simulink model "pipeline"  (Simulink 10.0)
settings: Solver=VariableStepAuto  StartTime=0.0  StopTime=10000*(1/2e7)  FixedStep=1e-9  RelTol=1e-3
values from neighbouring files (symbols this model uses):
  fsig = 13e6    (= 13000000)    [Pipeline_m.m]
  Ts = ts    (= 1e-08)    [Pipeline_m.m]
  vin_amp = vref*10^(-Vsig_dB/20)    (= 1.8)    [Pipeline_m.m]
settings Model: Creator=user  LastModifiedBy=benve
settings DataIOCC: SaveFormat=Dataset  ReturnWorkspaceOutputs=on
settings OptimizationCC: LifeSpan=auto
settings DebuggingCC: UnderspecifiedInitializationDetection=Simplified  MergeDetectMultiDrivingBlocksExec=error  SFUnexpectedBacktrackingDiag=error  SFNoUnconditionalDefaultTransitionDiag=error  SFExecutionAtInitializationDiag=warning  ArithmeticOperatorsInVariantConditions=error
settings HardwareCC: ProdBitPerPointer=64  ProdBitPerSizeT=64  ProdBitPerPtrDiffT=64  ProdLargestAtomicFloat=Float  ProdIntDivRoundTo=Zero  ProdEndianess=LittleEndian  ProdWordSize=64  ProdHWDeviceType=Intel->x86-64 (Windows64)
settings ModelReferenceCC: PropagateSignalLabelsOutOfModel=on
settings SFSimCC: SimUseLocalCustomCode=on
settings RTWCC: RTWUseLocalCustomCode=on
settings CodeAppCC: StateflowObjectComments=off
settings GRTTargetCC: TargetLangStandard=C99 (ISO)  CombineOutputUpdateFcns=on  GRTInterface=off
settings ConfigComp: CovMetricSettings=dwe  CovHtmlReporting=off  CovSaveCumulativeToWorkspaceVar=off  CovSaveSingleToWorkspaceVar=off

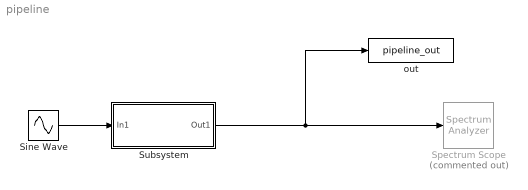
== system pipeline ==
  Sine Wave : Sin  Amplitude=vin_amp  Frequency=2*pi*fsig  SampleTime=Ts  VectorParams1D=off
  Spectrum Scope : SpectrumAnalyzer  Commented=on
  Subsystem : Subsystem  mask{Ts=Ts, vref=1.8}
      mask prompts: Ts "sampling time:"
  out : ToWorkspace  VariableName=pipeline_out  SampleTime=-1
      settings: Save2DSignal=2-D array (concatenate along first dimension)
  wires:
  Sine Wave/1 -> Subsystem/1(In1)
  Subsystem/1(Out1) -> out/1, Spectrum Scope/1

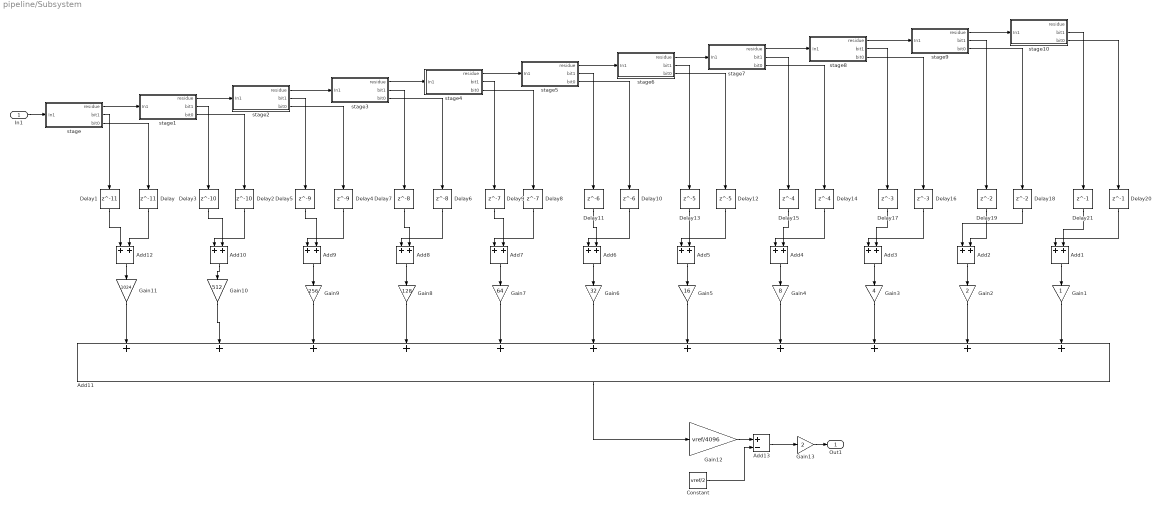
== system pipeline/Subsystem ==
  In1 : Inport
  Add{1..10,12} (11 alike) : Sum
  Add11 : Sum  Inputs=+++++++++++
  Add13 : Sum  Inputs=+-
  Constant : Constant  Value=vref/2
  Delay : Delay  DelayLength=11  SampleTime=Ts
  Delay1 : Delay  DelayLength=11  SampleTime=Ts
  Delay10 : Delay  DelayLength=6  SampleTime=Ts
  Delay11 : Delay  DelayLength=6  SampleTime=Ts
  Delay12 : Delay  DelayLength=5  SampleTime=Ts
  Delay13 : Delay  DelayLength=5  SampleTime=Ts
  Delay14 : Delay  DelayLength=4  SampleTime=Ts
  Delay15 : Delay  DelayLength=4  SampleTime=Ts
  Delay16 : Delay  DelayLength=3  SampleTime=Ts
  Delay17 : Delay  DelayLength=3  SampleTime=Ts
  Delay18 : Delay  SampleTime=Ts
  Delay19 : Delay  SampleTime=Ts
  Delay2 : Delay  DelayLength=10  SampleTime=Ts
  Delay20 : Delay  DelayLength=1  SampleTime=Ts
  Delay21 : Delay  DelayLength=1  SampleTime=Ts
  Delay3 : Delay  DelayLength=10  SampleTime=Ts
  Delay4 : Delay  DelayLength=9  SampleTime=Ts
  Delay5 : Delay  DelayLength=9  SampleTime=Ts
  Delay6 : Delay  DelayLength=8  SampleTime=Ts
  Delay7 : Delay  DelayLength=8  SampleTime=Ts
  Delay8 : Delay  DelayLength=7  SampleTime=Ts
  Delay9 : Delay  DelayLength=7  SampleTime=Ts
  Gain1 : Gain
  Gain10 : Gain  Gain=512
  Gain11 : Gain  Gain=1024
  Gain12 : Gain  Gain=vref/4096
  Gain13 : Gain  Gain=2
  Gain2 : Gain  Gain=2
  Gain3 : Gain  Gain=4
  Gain4 : Gain  Gain=8
  Gain5 : Gain  Gain=16
  Gain6 : Gain  Gain=32
  Gain7 : Gain  Gain=64
  Gain8 : Gain  Gain=128
  Gain9 : Gain  Gain=256
  stage : Subsystem
  stage1 : Subsystem
  stage10 : Subsystem
  stage2 : Subsystem
  stage3 : Subsystem
  stage4 : Subsystem
  stage5 : Subsystem
  stage6 : Subsystem
  stage7 : Subsystem
  stage8 : Subsystem
  stage9 : Subsystem
  Out1 : Outport  VectorParamsAs1DForOutWhenUnconnected=off
  wires:
  stage/1(residue) -> stage1/1(In1)
  stage1/1(residue) -> stage2/1(In1)
  In1/1 -> stage/1(In1)
  stage2/1(residue) -> stage3/1(In1)
  stage3/1(residue) -> stage4/1(In1)
  stage6/1(residue) -> stage7/1(In1)
  stage5/1(residue) -> stage6/1(In1)
  stage4/1(residue) -> stage5/1(In1)
  stage9/1(residue) -> stage10/1(In1)
  stage8/1(residue) -> stage9/1(In1)
  stage7/1(residue) -> stage8/1(In1)
  stage/2(bit1) -> Delay1/1
  stage/3(bit0) -> Delay/1
  stage1/3(bit0) -> Delay2/1
  stage1/2(bit1) -> Delay3/1
  stage2/3(bit0) -> Delay4/1
  stage2/2(bit1) -> Delay5/1
  stage3/2(bit1) -> Delay7/1
  stage3/3(bit0) -> Delay6/1
  stage4/3(bit0) -> Delay8/1
  stage4/2(bit1) -> Delay9/1
  stage5/3(bit0) -> Delay10/1
  stage5/2(bit1) -> Delay11/1
  stage6/2(bit1) -> Delay13/1
  stage6/3(bit0) -> Delay12/1
  stage7/3(bit0) -> Delay14/1
  stage7/2(bit1) -> Delay15/1
  stage8/3(bit0) -> Delay16/1
  stage8/2(bit1) -> Delay17/1
  stage9/2(bit1) -> Delay19/1
  stage9/3(bit0) -> Delay18/1
  stage10/2(bit1) -> Delay21/1
  stage10/3(bit0) -> Delay20/1
  Add1/1 -> Gain1/1
  Delay21/1 -> Add1/2
  Add2/1 -> Gain2/1
  Delay19/1 -> Add2/2
  Delay17/1 -> Add3/2
  Add3/1 -> Gain3/1
  Add4/1 -> Gain4/1
  Delay15/1 -> Add4/2
  Add5/1 -> Gain5/1
  Delay13/1 -> Add5/2
  Add6/1 -> Gain6/1
  Delay11/1 -> Add6/2
  Add7/1 -> Gain7/1
  Delay9/1 -> Add7/2
  Add8/1 -> Gain8/1
  Delay7/1 -> Add8/2
  Add9/1 -> Gain9/1
  Delay5/1 -> Add9/2
  Add10/1 -> Gain10/1
  Delay3/1 -> Add10/2
  Gain1/1 -> Add11/11
  Gain2/1 -> Add11/10
  Gain3/1 -> Add11/9
  Gain4/1 -> Add11/8
  Gain5/1 -> Add11/7
  Gain6/1 -> Add11/6
  Gain7/1 -> Add11/5
  Gain8/1 -> Add11/4
  Gain9/1 -> Add11/3
  Gain10/1 -> Add11/2
  Gain11/1 -> Add11/1
  Delay20/1 -> Add1/1
  Delay18/1 -> Add2/1
  Delay16/1 -> Add3/1
  Delay14/1 -> Add4/1
  Delay12/1 -> Add5/1
  Delay10/1 -> Add6/1
  Delay8/1 -> Add7/1
  Delay6/1 -> Add8/1
  Delay4/1 -> Add9/1
  Delay2/1 -> Add10/1
  Delay1/1 -> Add12/1
  Delay/1 -> Add12/2
  Add12/1 -> Gain11/1
  Add11/1 -> Gain12/1
  Gain12/1 -> Add13/1
  Add13/1 -> Gain13/1
  Constant/1 -> Add13/2
  Gain13/1 -> Out1/1

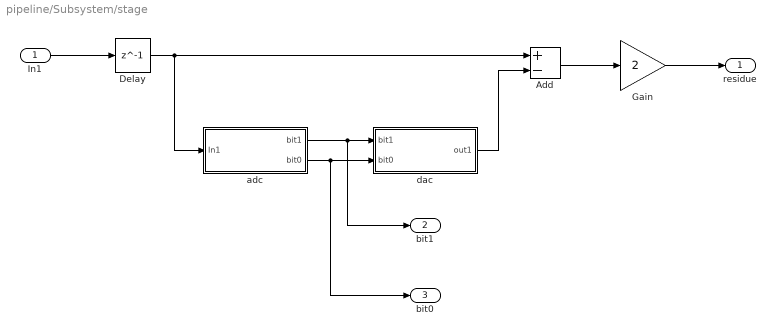
== system pipeline/Subsystem/stage ==
  In1 : Inport
  Add : Sum  Inputs=+-
  Delay : Delay  DelayLength=1  SampleTime=Ts
  Gain : Gain  Gain=2
  adc : Subsystem
  dac : Subsystem
  residue : Outport  VectorParamsAs1DForOutWhenUnconnected=off
  bit1 : Outport  Port=2  VectorParamsAs1DForOutWhenUnconnected=off
  bit0 : Outport  Port=3  VectorParamsAs1DForOutWhenUnconnected=off
  wires:
  adc/1(bit1) -> bit1/1, dac/1(bit1)
  dac/1(out1) -> Add/2
  Delay/1 -> adc/1(In1), Add/1
  Gain/1 -> residue/1
  Add/1 -> Gain/1
  In1/1 -> Delay/1
  adc/2(bit0) -> bit0/1, dac/2(bit0)

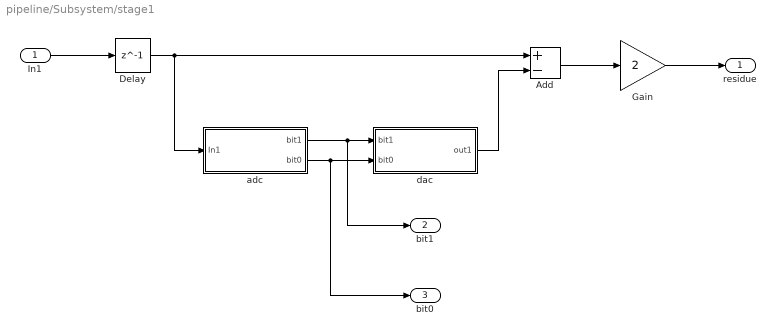
== system pipeline/Subsystem/stage1 ==
  In1 : Inport
  Add : Sum  Inputs=+-
  Delay : Delay  DelayLength=1  SampleTime=Ts
  Gain : Gain  Gain=2
  adc : Subsystem
  dac : Subsystem
  residue : Outport  VectorParamsAs1DForOutWhenUnconnected=off
  bit1 : Outport  Port=2  VectorParamsAs1DForOutWhenUnconnected=off
  bit0 : Outport  Port=3  VectorParamsAs1DForOutWhenUnconnected=off
  wires:
  adc/1(bit1) -> bit1/1, dac/1(bit1)
  dac/1(out1) -> Add/2
  Delay/1 -> adc/1(In1), Add/1
  Gain/1 -> residue/1
  Add/1 -> Gain/1
  In1/1 -> Delay/1
  adc/2(bit0) -> bit0/1, dac/2(bit0)

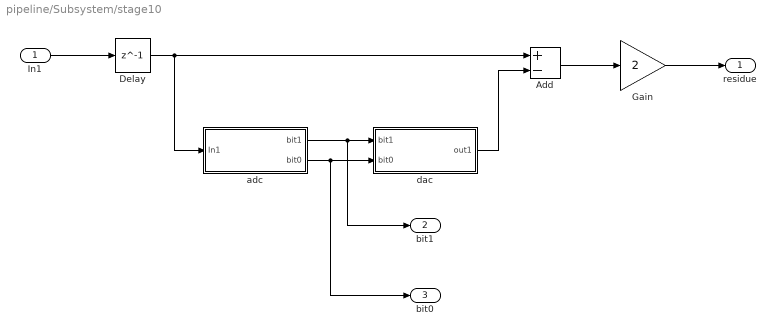
== system pipeline/Subsystem/stage10 ==
  In1 : Inport
  Add : Sum  Inputs=+-
  Delay : Delay  DelayLength=1  SampleTime=Ts
  Gain : Gain  Gain=2
  adc : Subsystem
  dac : Subsystem
  residue : Outport  VectorParamsAs1DForOutWhenUnconnected=off
  bit1 : Outport  Port=2  VectorParamsAs1DForOutWhenUnconnected=off
  bit0 : Outport  Port=3  VectorParamsAs1DForOutWhenUnconnected=off
  wires:
  adc/1(bit1) -> bit1/1, dac/1(bit1)
  dac/1(out1) -> Add/2
  Delay/1 -> adc/1(In1), Add/1
  Gain/1 -> residue/1
  Add/1 -> Gain/1
  In1/1 -> Delay/1
  adc/2(bit0) -> bit0/1, dac/2(bit0)

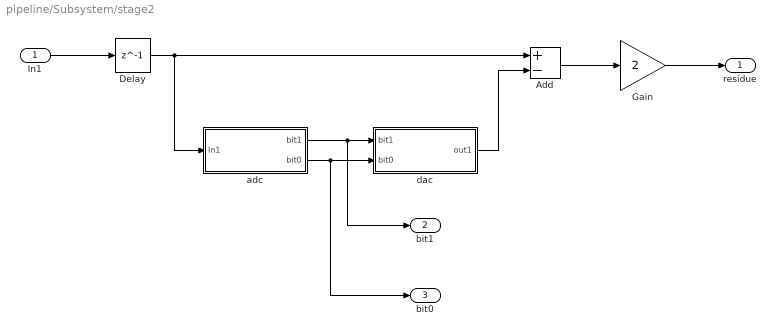
== system pipeline/Subsystem/stage2 ==
  In1 : Inport
  Add : Sum  Inputs=+-
  Delay : Delay  DelayLength=1  SampleTime=Ts
  Gain : Gain  Gain=2
  adc : Subsystem
  dac : Subsystem
  residue : Outport  VectorParamsAs1DForOutWhenUnconnected=off
  bit1 : Outport  Port=2  VectorParamsAs1DForOutWhenUnconnected=off
  bit0 : Outport  Port=3  VectorParamsAs1DForOutWhenUnconnected=off
  wires:
  adc/1(bit1) -> bit1/1, dac/1(bit1)
  dac/1(out1) -> Add/2
  Delay/1 -> adc/1(In1), Add/1
  Gain/1 -> residue/1
  Add/1 -> Gain/1
  In1/1 -> Delay/1
  adc/2(bit0) -> bit0/1, dac/2(bit0)

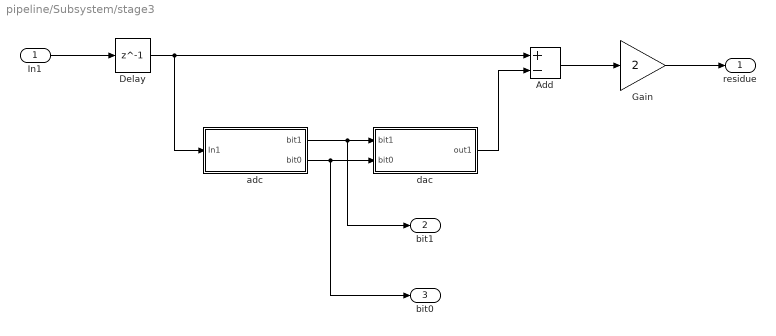
== system pipeline/Subsystem/stage3 ==
  In1 : Inport
  Add : Sum  Inputs=+-
  Delay : Delay  DelayLength=1  SampleTime=Ts
  Gain : Gain  Gain=2
  adc : Subsystem
  dac : Subsystem
  residue : Outport  VectorParamsAs1DForOutWhenUnconnected=off
  bit1 : Outport  Port=2  VectorParamsAs1DForOutWhenUnconnected=off
  bit0 : Outport  Port=3  VectorParamsAs1DForOutWhenUnconnected=off
  wires:
  adc/1(bit1) -> bit1/1, dac/1(bit1)
  dac/1(out1) -> Add/2
  Delay/1 -> adc/1(In1), Add/1
  Gain/1 -> residue/1
  Add/1 -> Gain/1
  In1/1 -> Delay/1
  adc/2(bit0) -> bit0/1, dac/2(bit0)

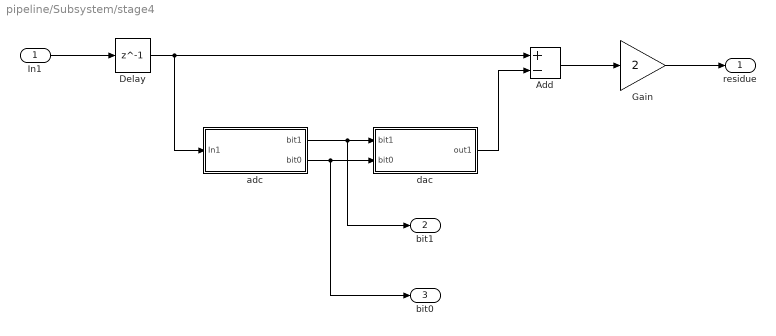
== system pipeline/Subsystem/stage4 ==
  In1 : Inport
  Add : Sum  Inputs=+-
  Delay : Delay  DelayLength=1  SampleTime=Ts
  Gain : Gain  Gain=2
  adc : Subsystem
  dac : Subsystem
  residue : Outport  VectorParamsAs1DForOutWhenUnconnected=off
  bit1 : Outport  Port=2  VectorParamsAs1DForOutWhenUnconnected=off
  bit0 : Outport  Port=3  VectorParamsAs1DForOutWhenUnconnected=off
  wires:
  adc/1(bit1) -> bit1/1, dac/1(bit1)
  dac/1(out1) -> Add/2
  Delay/1 -> adc/1(In1), Add/1
  Gain/1 -> residue/1
  Add/1 -> Gain/1
  In1/1 -> Delay/1
  adc/2(bit0) -> bit0/1, dac/2(bit0)

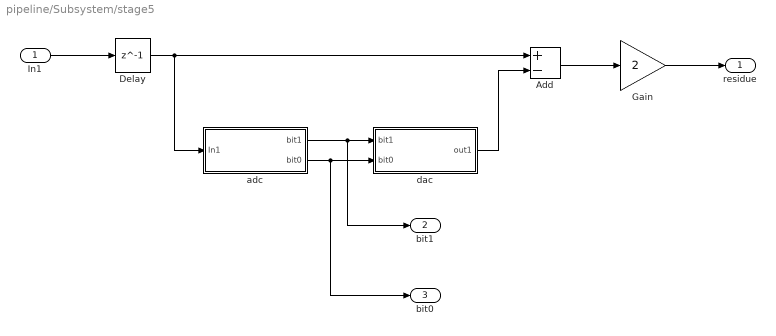
== system pipeline/Subsystem/stage5 ==
  In1 : Inport
  Add : Sum  Inputs=+-
  Delay : Delay  DelayLength=1  SampleTime=Ts
  Gain : Gain  Gain=2
  adc : Subsystem
  dac : Subsystem
  residue : Outport  VectorParamsAs1DForOutWhenUnconnected=off
  bit1 : Outport  Port=2  VectorParamsAs1DForOutWhenUnconnected=off
  bit0 : Outport  Port=3  VectorParamsAs1DForOutWhenUnconnected=off
  wires:
  adc/1(bit1) -> bit1/1, dac/1(bit1)
  dac/1(out1) -> Add/2
  Delay/1 -> adc/1(In1), Add/1
  Gain/1 -> residue/1
  Add/1 -> Gain/1
  In1/1 -> Delay/1
  adc/2(bit0) -> bit0/1, dac/2(bit0)

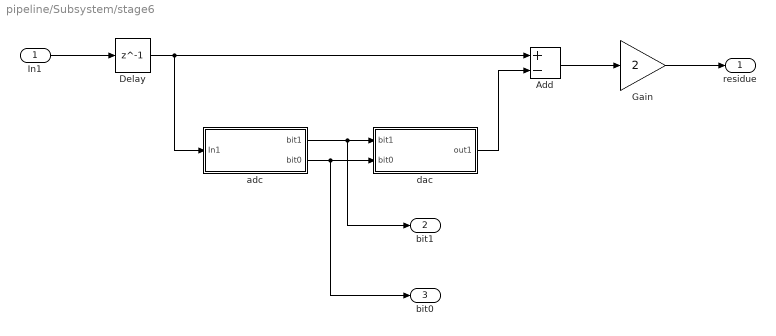
== system pipeline/Subsystem/stage6 ==
  In1 : Inport
  Add : Sum  Inputs=+-
  Delay : Delay  DelayLength=1  SampleTime=Ts
  Gain : Gain  Gain=2
  adc : Subsystem
  dac : Subsystem
  residue : Outport  VectorParamsAs1DForOutWhenUnconnected=off
  bit1 : Outport  Port=2  VectorParamsAs1DForOutWhenUnconnected=off
  bit0 : Outport  Port=3  VectorParamsAs1DForOutWhenUnconnected=off
  wires:
  adc/1(bit1) -> bit1/1, dac/1(bit1)
  dac/1(out1) -> Add/2
  Delay/1 -> adc/1(In1), Add/1
  Gain/1 -> residue/1
  Add/1 -> Gain/1
  In1/1 -> Delay/1
  adc/2(bit0) -> bit0/1, dac/2(bit0)

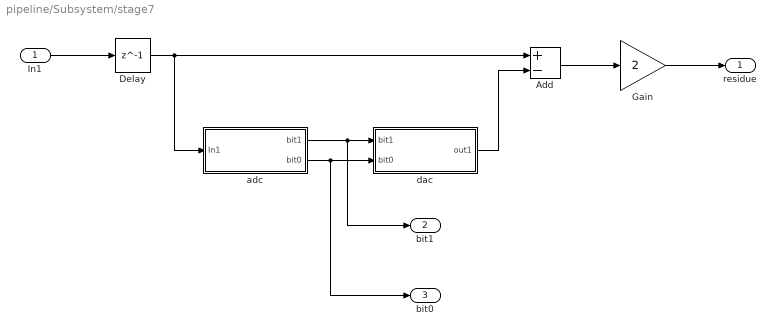
== system pipeline/Subsystem/stage7 ==
  In1 : Inport
  Add : Sum  Inputs=+-
  Delay : Delay  DelayLength=1  SampleTime=Ts
  Gain : Gain  Gain=2
  adc : Subsystem
  dac : Subsystem
  residue : Outport  VectorParamsAs1DForOutWhenUnconnected=off
  bit1 : Outport  Port=2  VectorParamsAs1DForOutWhenUnconnected=off
  bit0 : Outport  Port=3  VectorParamsAs1DForOutWhenUnconnected=off
  wires:
  adc/1(bit1) -> bit1/1, dac/1(bit1)
  dac/1(out1) -> Add/2
  Delay/1 -> adc/1(In1), Add/1
  Gain/1 -> residue/1
  Add/1 -> Gain/1
  In1/1 -> Delay/1
  adc/2(bit0) -> bit0/1, dac/2(bit0)

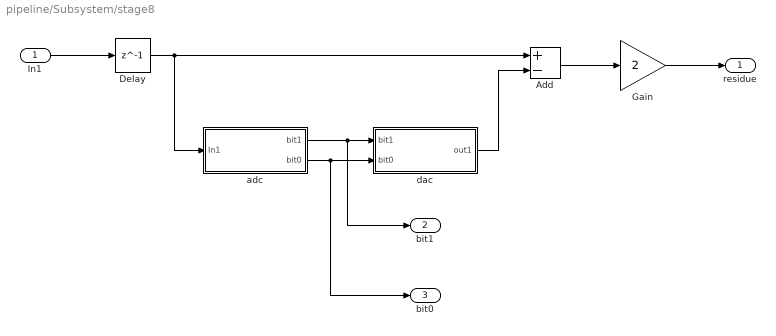
== system pipeline/Subsystem/stage8 ==
  In1 : Inport
  Add : Sum  Inputs=+-
  Delay : Delay  DelayLength=1  SampleTime=Ts
  Gain : Gain  Gain=2
  adc : Subsystem
  dac : Subsystem
  residue : Outport  VectorParamsAs1DForOutWhenUnconnected=off
  bit1 : Outport  Port=2  VectorParamsAs1DForOutWhenUnconnected=off
  bit0 : Outport  Port=3  VectorParamsAs1DForOutWhenUnconnected=off
  wires:
  adc/1(bit1) -> bit1/1, dac/1(bit1)
  dac/1(out1) -> Add/2
  Delay/1 -> adc/1(In1), Add/1
  Gain/1 -> residue/1
  Add/1 -> Gain/1
  In1/1 -> Delay/1
  adc/2(bit0) -> bit0/1, dac/2(bit0)

== system pipeline/Subsystem/stage9 ==
  In1 : Inport
  Add : Sum  Inputs=+-
  Delay : Delay  DelayLength=1  SampleTime=Ts
  Gain : Gain  Gain=2
  adc : Subsystem
  dac : Subsystem
  residue : Outport  VectorParamsAs1DForOutWhenUnconnected=off
  bit1 : Outport  Port=2  VectorParamsAs1DForOutWhenUnconnected=off
  bit0 : Outport  Port=3  VectorParamsAs1DForOutWhenUnconnected=off
  wires:
  adc/1(bit1) -> bit1/1, dac/1(bit1)
  dac/1(out1) -> Add/2
  Delay/1 -> adc/1(In1), Add/1
  Gain/1 -> residue/1
  Add/1 -> Gain/1
  In1/1 -> Delay/1
  adc/2(bit0) -> bit0/1, dac/2(bit0)

== system pipeline/Subsystem/stage/adc ==
  In1 : Inport
  Add : Sum  Inputs=+-
  Add1 : Sum  Inputs=+-
  Constant : Constant  Value=vref/3
  Constant1 : Constant  Value=-vref/3
  Relay : Relay  OnSwitchValue=0  OffSwitchValue=0
  Relay1 : Relay  OnSwitchValue=0  OffSwitchValue=0
  bit1 : Outport  VectorParamsAs1DForOutWhenUnconnected=off
  bit0 : Outport  Port=2  VectorParamsAs1DForOutWhenUnconnected=off
  wires:
  In1/1 -> Add1/1, Add/1
  Constant/1 -> Add/2
  Constant1/1 -> Add1/2
  Add/1 -> Relay/1
  Add1/1 -> Relay1/1
  Relay/1 -> bit1/1
  Relay1/1 -> bit0/1

== system pipeline/Subsystem/stage/dac ==
  bit1 : Inport
  bit0 : Inport  Port=2
  Add : Sum
  Constant : Constant  Value=vref/2
  Constant1 : Constant  Value=-vref/2
  Constant2 : Constant  Value=0
  Switch : Switch  Criteria=u2 > Threshold
  Switch1 : Switch  Criteria=u2 > Threshold
  out1 : Outport  VectorParamsAs1DForOutWhenUnconnected=off
  wires:
  bit1/1 -> Switch/2
  bit0/1 -> Switch1/2
  Constant1/1 -> Switch1/3
  Constant/1 -> Switch/1
  Constant2/1 -> Switch/3, Switch1/1
  Switch1/1 -> Add/2
  Switch/1 -> Add/1
  Add/1 -> out1/1

== system pipeline/Subsystem/stage1/adc ==
  In1 : Inport
  Add : Sum  Inputs=+-
  Add1 : Sum  Inputs=+-
  Constant : Constant  Value=vref/3
  Constant1 : Constant  Value=-vref/3
  Relay : Relay  OnSwitchValue=0  OffSwitchValue=0
  Relay1 : Relay  OnSwitchValue=0  OffSwitchValue=0
  bit1 : Outport  VectorParamsAs1DForOutWhenUnconnected=off
  bit0 : Outport  Port=2  VectorParamsAs1DForOutWhenUnconnected=off
  wires:
  In1/1 -> Add1/1, Add/1
  Constant/1 -> Add/2
  Constant1/1 -> Add1/2
  Add/1 -> Relay/1
  Add1/1 -> Relay1/1
  Relay/1 -> bit1/1
  Relay1/1 -> bit0/1

== system pipeline/Subsystem/stage1/dac ==
  bit1 : Inport
  bit0 : Inport  Port=2
  Add : Sum
  Constant : Constant  Value=vref/2
  Constant1 : Constant  Value=-vref/2
  Constant2 : Constant  Value=0
  Switch : Switch  Criteria=u2 > Threshold
  Switch1 : Switch  Criteria=u2 > Threshold
  out1 : Outport  VectorParamsAs1DForOutWhenUnconnected=off
  wires:
  bit1/1 -> Switch/2
  bit0/1 -> Switch1/2
  Constant1/1 -> Switch1/3
  Constant/1 -> Switch/1
  Constant2/1 -> Switch/3, Switch1/1
  Switch1/1 -> Add/2
  Switch/1 -> Add/1
  Add/1 -> out1/1

== system pipeline/Subsystem/stage10/adc ==
  In1 : Inport
  Add : Sum  Inputs=+-
  Add1 : Sum  Inputs=+-
  Constant : Constant  Value=vref/3
  Constant1 : Constant  Value=-vref/3
  Relay : Relay  OnSwitchValue=0  OffSwitchValue=0
  Relay1 : Relay  OnSwitchValue=0  OffSwitchValue=0
  bit1 : Outport  VectorParamsAs1DForOutWhenUnconnected=off
  bit0 : Outport  Port=2  VectorParamsAs1DForOutWhenUnconnected=off
  wires:
  In1/1 -> Add1/1, Add/1
  Constant/1 -> Add/2
  Constant1/1 -> Add1/2
  Add/1 -> Relay/1
  Add1/1 -> Relay1/1
  Relay/1 -> bit1/1
  Relay1/1 -> bit0/1

== system pipeline/Subsystem/stage10/dac ==
  bit1 : Inport
  bit0 : Inport  Port=2
  Add : Sum
  Constant : Constant  Value=vref/2
  Constant1 : Constant  Value=-vref/2
  Constant2 : Constant  Value=0
  Switch : Switch  Criteria=u2 > Threshold
  Switch1 : Switch  Criteria=u2 > Threshold
  out1 : Outport  VectorParamsAs1DForOutWhenUnconnected=off
  wires:
  bit1/1 -> Switch/2
  bit0/1 -> Switch1/2
  Constant1/1 -> Switch1/3
  Constant/1 -> Switch/1
  Constant2/1 -> Switch/3, Switch1/1
  Switch1/1 -> Add/2
  Switch/1 -> Add/1
  Add/1 -> out1/1

== system pipeline/Subsystem/stage2/adc ==
  In1 : Inport
  Add : Sum  Inputs=+-
  Add1 : Sum  Inputs=+-
  Constant : Constant  Value=vref/3
  Constant1 : Constant  Value=-vref/3
  Relay : Relay  OnSwitchValue=0  OffSwitchValue=0
  Relay1 : Relay  OnSwitchValue=0  OffSwitchValue=0
  bit1 : Outport  VectorParamsAs1DForOutWhenUnconnected=off
  bit0 : Outport  Port=2  VectorParamsAs1DForOutWhenUnconnected=off
  wires:
  In1/1 -> Add1/1, Add/1
  Constant/1 -> Add/2
  Constant1/1 -> Add1/2
  Add/1 -> Relay/1
  Add1/1 -> Relay1/1
  Relay/1 -> bit1/1
  Relay1/1 -> bit0/1

== system pipeline/Subsystem/stage2/dac ==
  bit1 : Inport
  bit0 : Inport  Port=2
  Add : Sum
  Constant : Constant  Value=vref/2
  Constant1 : Constant  Value=-vref/2
  Constant2 : Constant  Value=0
  Switch : Switch  Criteria=u2 > Threshold
  Switch1 : Switch  Criteria=u2 > Threshold
  out1 : Outport  VectorParamsAs1DForOutWhenUnconnected=off
  wires:
  bit1/1 -> Switch/2
  bit0/1 -> Switch1/2
  Constant1/1 -> Switch1/3
  Constant/1 -> Switch/1
  Constant2/1 -> Switch/3, Switch1/1
  Switch1/1 -> Add/2
  Switch/1 -> Add/1
  Add/1 -> out1/1

== system pipeline/Subsystem/stage3/adc ==
  In1 : Inport
  Add : Sum  Inputs=+-
  Add1 : Sum  Inputs=+-
  Constant : Constant  Value=vref/3
  Constant1 : Constant  Value=-vref/3
  Relay : Relay  OnSwitchValue=0  OffSwitchValue=0
  Relay1 : Relay  OnSwitchValue=0  OffSwitchValue=0
  bit1 : Outport  VectorParamsAs1DForOutWhenUnconnected=off
  bit0 : Outport  Port=2  VectorParamsAs1DForOutWhenUnconnected=off
  wires:
  In1/1 -> Add1/1, Add/1
  Constant/1 -> Add/2
  Constant1/1 -> Add1/2
  Add/1 -> Relay/1
  Add1/1 -> Relay1/1
  Relay/1 -> bit1/1
  Relay1/1 -> bit0/1

== system pipeline/Subsystem/stage3/dac ==
  bit1 : Inport
  bit0 : Inport  Port=2
  Add : Sum
  Constant : Constant  Value=vref/2
  Constant1 : Constant  Value=-vref/2
  Constant2 : Constant  Value=0
  Switch : Switch  Criteria=u2 > Threshold
  Switch1 : Switch  Criteria=u2 > Threshold
  out1 : Outport  VectorParamsAs1DForOutWhenUnconnected=off
  wires:
  bit1/1 -> Switch/2
  bit0/1 -> Switch1/2
  Constant1/1 -> Switch1/3
  Constant/1 -> Switch/1
  Constant2/1 -> Switch/3, Switch1/1
  Switch1/1 -> Add/2
  Switch/1 -> Add/1
  Add/1 -> out1/1

== system pipeline/Subsystem/stage4/adc ==
  In1 : Inport
  Add : Sum  Inputs=+-
  Add1 : Sum  Inputs=+-
  Constant : Constant  Value=vref/3
  Constant1 : Constant  Value=-vref/3
  Relay : Relay  OnSwitchValue=0  OffSwitchValue=0
  Relay1 : Relay  OnSwitchValue=0  OffSwitchValue=0
  bit1 : Outport  VectorParamsAs1DForOutWhenUnconnected=off
  bit0 : Outport  Port=2  VectorParamsAs1DForOutWhenUnconnected=off
  wires:
  In1/1 -> Add1/1, Add/1
  Constant/1 -> Add/2
  Constant1/1 -> Add1/2
  Add/1 -> Relay/1
  Add1/1 -> Relay1/1
  Relay/1 -> bit1/1
  Relay1/1 -> bit0/1

== system pipeline/Subsystem/stage4/dac ==
  bit1 : Inport
  bit0 : Inport  Port=2
  Add : Sum
  Constant : Constant  Value=vref/2
  Constant1 : Constant  Value=-vref/2
  Constant2 : Constant  Value=0
  Switch : Switch  Criteria=u2 > Threshold
  Switch1 : Switch  Criteria=u2 > Threshold
  out1 : Outport  VectorParamsAs1DForOutWhenUnconnected=off
  wires:
  bit1/1 -> Switch/2
  bit0/1 -> Switch1/2
  Constant1/1 -> Switch1/3
  Constant/1 -> Switch/1
  Constant2/1 -> Switch/3, Switch1/1
  Switch1/1 -> Add/2
  Switch/1 -> Add/1
  Add/1 -> out1/1

== system pipeline/Subsystem/stage5/adc ==
  In1 : Inport
  Add : Sum  Inputs=+-
  Add1 : Sum  Inputs=+-
  Constant : Constant  Value=vref/3
  Constant1 : Constant  Value=-vref/3
  Relay : Relay  OnSwitchValue=0  OffSwitchValue=0
  Relay1 : Relay  OnSwitchValue=0  OffSwitchValue=0
  bit1 : Outport  VectorParamsAs1DForOutWhenUnconnected=off
  bit0 : Outport  Port=2  VectorParamsAs1DForOutWhenUnconnected=off
  wires:
  In1/1 -> Add1/1, Add/1
  Constant/1 -> Add/2
  Constant1/1 -> Add1/2
  Add/1 -> Relay/1
  Add1/1 -> Relay1/1
  Relay/1 -> bit1/1
  Relay1/1 -> bit0/1

== system pipeline/Subsystem/stage5/dac ==
  bit1 : Inport
  bit0 : Inport  Port=2
  Add : Sum
  Constant : Constant  Value=vref/2
  Constant1 : Constant  Value=-vref/2
  Constant2 : Constant  Value=0
  Switch : Switch  Criteria=u2 > Threshold
  Switch1 : Switch  Criteria=u2 > Threshold
  out1 : Outport  VectorParamsAs1DForOutWhenUnconnected=off
  wires:
  bit1/1 -> Switch/2
  bit0/1 -> Switch1/2
  Constant1/1 -> Switch1/3
  Constant/1 -> Switch/1
  Constant2/1 -> Switch/3, Switch1/1
  Switch1/1 -> Add/2
  Switch/1 -> Add/1
  Add/1 -> out1/1

== system pipeline/Subsystem/stage6/adc ==
  In1 : Inport
  Add : Sum  Inputs=+-
  Add1 : Sum  Inputs=+-
  Constant : Constant  Value=vref/3
  Constant1 : Constant  Value=-vref/3
  Relay : Relay  OnSwitchValue=0  OffSwitchValue=0
  Relay1 : Relay  OnSwitchValue=0  OffSwitchValue=0
  bit1 : Outport  VectorParamsAs1DForOutWhenUnconnected=off
  bit0 : Outport  Port=2  VectorParamsAs1DForOutWhenUnconnected=off
  wires:
  In1/1 -> Add1/1, Add/1
  Constant/1 -> Add/2
  Constant1/1 -> Add1/2
  Add/1 -> Relay/1
  Add1/1 -> Relay1/1
  Relay/1 -> bit1/1
  Relay1/1 -> bit0/1

== system pipeline/Subsystem/stage6/dac ==
  bit1 : Inport
  bit0 : Inport  Port=2
  Add : Sum
  Constant : Constant  Value=vref/2
  Constant1 : Constant  Value=-vref/2
  Constant2 : Constant  Value=0
  Switch : Switch  Criteria=u2 > Threshold
  Switch1 : Switch  Criteria=u2 > Threshold
  out1 : Outport  VectorParamsAs1DForOutWhenUnconnected=off
  wires:
  bit1/1 -> Switch/2
  bit0/1 -> Switch1/2
  Constant1/1 -> Switch1/3
  Constant/1 -> Switch/1
  Constant2/1 -> Switch/3, Switch1/1
  Switch1/1 -> Add/2
  Switch/1 -> Add/1
  Add/1 -> out1/1

== system pipeline/Subsystem/stage7/adc ==
  In1 : Inport
  Add : Sum  Inputs=+-
  Add1 : Sum  Inputs=+-
  Constant : Constant  Value=vref/3
  Constant1 : Constant  Value=-vref/3
  Relay : Relay  OnSwitchValue=0  OffSwitchValue=0
  Relay1 : Relay  OnSwitchValue=0  OffSwitchValue=0
  bit1 : Outport  VectorParamsAs1DForOutWhenUnconnected=off
  bit0 : Outport  Port=2  VectorParamsAs1DForOutWhenUnconnected=off
  wires:
  In1/1 -> Add1/1, Add/1
  Constant/1 -> Add/2
  Constant1/1 -> Add1/2
  Add/1 -> Relay/1
  Add1/1 -> Relay1/1
  Relay/1 -> bit1/1
  Relay1/1 -> bit0/1

== system pipeline/Subsystem/stage7/dac ==
  bit1 : Inport
  bit0 : Inport  Port=2
  Add : Sum
  Constant : Constant  Value=vref/2
  Constant1 : Constant  Value=-vref/2
  Constant2 : Constant  Value=0
  Switch : Switch  Criteria=u2 > Threshold
  Switch1 : Switch  Criteria=u2 > Threshold
  out1 : Outport  VectorParamsAs1DForOutWhenUnconnected=off
  wires:
  bit1/1 -> Switch/2
  bit0/1 -> Switch1/2
  Constant1/1 -> Switch1/3
  Constant/1 -> Switch/1
  Constant2/1 -> Switch/3, Switch1/1
  Switch1/1 -> Add/2
  Switch/1 -> Add/1
  Add/1 -> out1/1

== system pipeline/Subsystem/stage8/adc ==
  In1 : Inport
  Add : Sum  Inputs=+-
  Add1 : Sum  Inputs=+-
  Constant : Constant  Value=vref/3
  Constant1 : Constant  Value=-vref/3
  Relay : Relay  OnSwitchValue=0  OffSwitchValue=0
  Relay1 : Relay  OnSwitchValue=0  OffSwitchValue=0
  bit1 : Outport  VectorParamsAs1DForOutWhenUnconnected=off
  bit0 : Outport  Port=2  VectorParamsAs1DForOutWhenUnconnected=off
  wires:
  In1/1 -> Add1/1, Add/1
  Constant/1 -> Add/2
  Constant1/1 -> Add1/2
  Add/1 -> Relay/1
  Add1/1 -> Relay1/1
  Relay/1 -> bit1/1
  Relay1/1 -> bit0/1

== system pipeline/Subsystem/stage8/dac ==
  bit1 : Inport
  bit0 : Inport  Port=2
  Add : Sum
  Constant : Constant  Value=vref/2
  Constant1 : Constant  Value=-vref/2
  Constant2 : Constant  Value=0
  Switch : Switch  Criteria=u2 > Threshold
  Switch1 : Switch  Criteria=u2 > Threshold
  out1 : Outport  VectorParamsAs1DForOutWhenUnconnected=off
  wires:
  bit1/1 -> Switch/2
  bit0/1 -> Switch1/2
  Constant1/1 -> Switch1/3
  Constant/1 -> Switch/1
  Constant2/1 -> Switch/3, Switch1/1
  Switch1/1 -> Add/2
  Switch/1 -> Add/1
  Add/1 -> out1/1

== system pipeline/Subsystem/stage9/adc ==
  In1 : Inport
  Add : Sum  Inputs=+-
  Add1 : Sum  Inputs=+-
  Constant : Constant  Value=vref/3
  Constant1 : Constant  Value=-vref/3
  Relay : Relay  OnSwitchValue=0  OffSwitchValue=0
  Relay1 : Relay  OnSwitchValue=0  OffSwitchValue=0
  bit1 : Outport  VectorParamsAs1DForOutWhenUnconnected=off
  bit0 : Outport  Port=2  VectorParamsAs1DForOutWhenUnconnected=off
  wires:
  In1/1 -> Add1/1, Add/1
  Constant/1 -> Add/2
  Constant1/1 -> Add1/2
  Add/1 -> Relay/1
  Add1/1 -> Relay1/1
  Relay/1 -> bit1/1
  Relay1/1 -> bit0/1

== system pipeline/Subsystem/stage9/dac ==
  bit1 : Inport
  bit0 : Inport  Port=2
  Add : Sum
  Constant : Constant  Value=vref/2
  Constant1 : Constant  Value=-vref/2
  Constant2 : Constant  Value=0
  Switch : Switch  Criteria=u2 > Threshold
  Switch1 : Switch  Criteria=u2 > Threshold
  out1 : Outport  VectorParamsAs1DForOutWhenUnconnected=off
  wires:
  bit1/1 -> Switch/2
  bit0/1 -> Switch1/2
  Constant1/1 -> Switch1/3
  Constant/1 -> Switch/1
  Constant2/1 -> Switch/3, Switch1/1
  Switch1/1 -> Add/2
  Switch/1 -> Add/1
  Add/1 -> out1/1
